simulink model "FLL"  (R2018a)
settings: Solver=FixedStepAuto  StartTime=0.0  StopTime=2  FixedStep=1e-4  RelTol=1e-3
InitFcn:
  | gamma = 0.5
  | k = 1.414
undefined symbols (not defined in the file or in its folder): DiscIntNeverNeededParam
settings Model: Creator=donghao  LastModifiedBy=donghao
settings SolverCC: AlgebraicLoopSolver=LineSearch

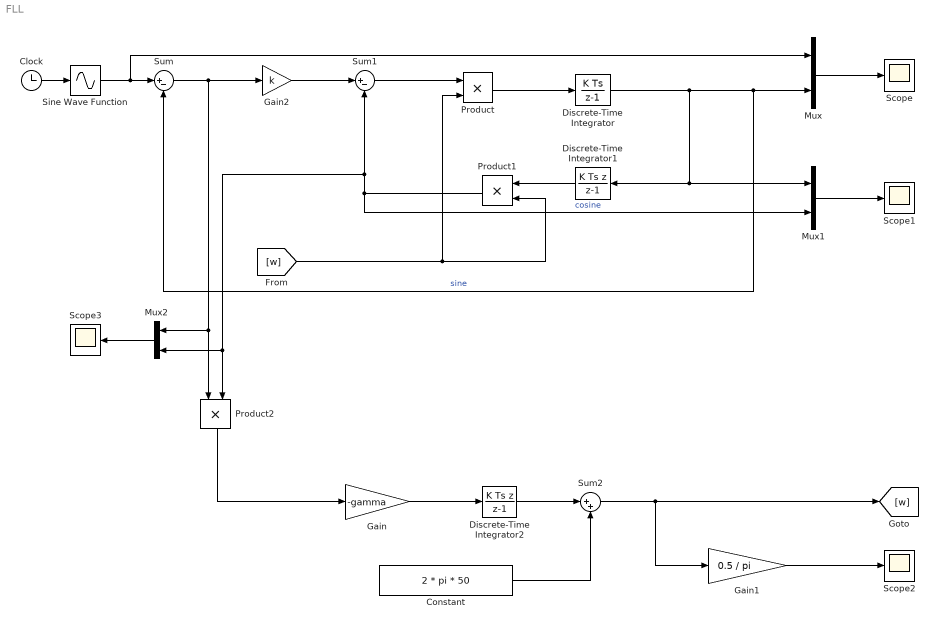
== system FLL ==
  Clock : Clock
  Constant : Constant  Value=2 * pi * 50
  Discrete-Time Integrator : DiscreteIntegrator  gainval=1  SampleTime=1e-4  ICPrevOutput=DiscIntNeverNeededParam  ICPrevScaledInput=DiscIntNeverNeededParam
  Discrete-Time Integrator1 : DiscreteIntegrator  IntegratorMethod=Integration: Backward Euler  gainval=1  SampleTime=1e-4  ICPrevOutput=DiscIntNeverNeededParam  ICPrevScaledInput=DiscIntNeverNeededParam
  Discrete-Time Integrator2 : DiscreteIntegrator  IntegratorMethod=Integration: Backward Euler  gainval=1  SampleTime=1e-4  ICPrevOutput=DiscIntNeverNeededParam  ICPrevScaledInput=DiscIntNeverNeededParam
  Gain : Gain  Gain=-gamma
  Gain1 : Gain  Gain=0.5 / pi
  Gain2 : Gain  Gain=k
  Mux : Mux  Inputs=2
  Mux1 : Mux  Inputs=2
  Mux2 : Mux  Inputs=2
  Product : Product
  Product1 : Product
  Product2 : Product
  Scope{,1..3} (4 alike) : Scope
  Sine Wave Function : Sin  TimeSource=Use external signal  Amplitude=311  Frequency=50 * 2 * pi  Phase=1.5  SampleTime=0
  Sum : Sum  Inputs=|+-
  Sum1 : Sum  Inputs=|+-
  Sum2 : Sum  Inputs=|++
  wires:
  Clock/1 -> Sine Wave Function/1
  Sum/1 -> Mux2/1, Product2/1, Gain2/1
  Sum1/1 -> Product/1
  Product/1 -> Discrete-Time Integrator/1
  Discrete-Time Integrator/1 -> Mux1/1, Discrete-Time Integrator1/1, Mux/2, Sum/2  "sine"
  Discrete-Time Integrator1/1 -> Product1/1
  Product1/1 -> Mux1/2, Mux2/2, Product2/2, Sum1/2  "cosine"
  [w] -> Product1/2, Product/2
  Mux/1 -> Scope/1
  Mux1/1 -> Scope1/1
  Sine Wave Function/1 -> Mux/1, Sum/1
  Product2/1 -> Gain/1
  Gain/1 -> Discrete-Time Integrator2/1
  Discrete-Time Integrator2/1 -> Sum2/1
  Constant/1 -> Sum2/2
  Sum2/1 -> Gain1/1, [w]
  Gain1/1 -> Scope2/1
  Gain2/1 -> Sum1/1
  Mux2/1 -> Scope3/1
